simulink model "p4_model"  (R2025b)
settings: Solver=VariableStepAuto  StartTime=0.0  StopTime=10.0  RelTol=1e-3
undefined symbols (not defined in the file or in its folder): carData, datBat, datCar, datMotor
libraries: autolibshared x1, slpidlib x1
(part 3 of 3)

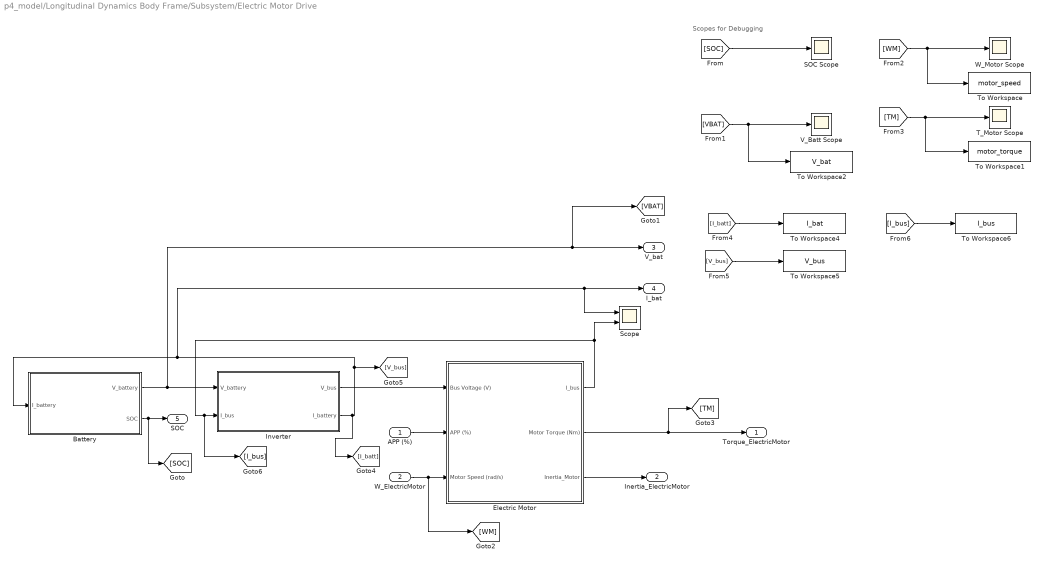
== system p4_model/Longitudinal Dynamics Body Frame/Subsystem/Electric Motor Drive ==
  note: Scopes for Debugging
  APP (%) : Inport
  W_ElectricMotor : Inport  Port=2
  Battery : Subsystem
  Electric Motor : Subsystem
  Inverter : Subsystem
  SOC Scope : Scope
      settings: ActiveDisplayYMinimum=0.79068  ActiveDisplayYMaximum=0.80103  DataLoggingVariableName=ScopeData7
  Scope : Scope  NumInputPorts=2
      settings: ActiveDisplayYMinimum=-92.41521  ActiveDisplayYMaximum=118.26537  DataLoggingVariableName=ScopeData2
  T_Motor Scope : Scope
      settings: ActiveDisplayYMinimum=-92.74121  ActiveDisplayYMaximum=115.47111  DataLoggingVariableName=ScopeData10
  To Workspace : ToWorkspace  VariableName=motor_speed  SaveFormat=Timeseries  SampleTime=-1
  To Workspace1 : ToWorkspace  VariableName=motor_torque  SaveFormat=Timeseries  SampleTime=-1
  To Workspace2 : ToWorkspace  VariableName=V_bat  SaveFormat=Timeseries  SampleTime=-1
  To Workspace4 : ToWorkspace  VariableName=I_bat  SaveFormat=Timeseries  SampleTime=-1
  To Workspace5 : ToWorkspace  VariableName=V_bus  SaveFormat=Timeseries  SampleTime=-1
  To Workspace6 : ToWorkspace  VariableName=I_bus  SaveFormat=Timeseries  SampleTime=-1
  V_Batt Scope : Scope
      settings: ActiveDisplayYMinimum=354.15627  ActiveDisplayYMaximum=391.49042  DataLoggingVariableName=ScopeData8
  W_Motor Scope : Scope
      settings: ActiveDisplayYMinimum=-83.74997  ActiveDisplayYMaximum=695.87961  DataLoggingVariableName=ScopeData9
  Torque_ElectricMotor : Outport
  Inertia_ElectricMotor : Outport  Port=2
  V_bat : Outport  Port=3
  I_bat : Outport  Port=4
  SOC : Outport  Port=5
  wires:
  APP (%)/1 -> Electric Motor/2(APP (%))
  W_ElectricMotor/1 -> [WM], Electric Motor/3(Motor Speed (rad/s))
  Electric Motor/3(Inertia_Motor) -> Inertia_ElectricMotor/1
  Inverter/1(V_bus) -> Electric Motor/1(Bus Voltage (V))
  Inverter/2(I_battery) -> [I_batt], Scope/1, I_bat/1, Battery/1(I_battery), [V_bus]
  Electric Motor/1(I_bus) -> Scope/2, [I_bus], Inverter/2(I_bus)
  [SOC] -> SOC Scope/1
  [VBAT] -> To Workspace2/1, V_Batt Scope/1
  [WM] -> To Workspace/1, W_Motor Scope/1
  [TM] -> To Workspace1/1, T_Motor Scope/1
  Battery/1(V_battery) -> [VBAT], V_bat/1, Inverter/1(V_battery)
  Electric Motor/2(Motor Torque (Nm)) -> [TM], Torque_ElectricMotor/1
  Battery/2(SOC) -> [SOC], SOC/1
  [I_batt] -> To Workspace4/1
  [V_bus] -> To Workspace5/1
  [I_bus] -> To Workspace6/1

== system p4_model/Longitudinal Dynamics Body Frame/Vehicle/vehicleDragForce ==
  vel : Inport
  Drag Force : MATLAB Function  TreatAsAtomicUnit=on
  To Workspace : ToWorkspace  VariableName=Faero  SaveFormat=Timeseries  SampleTime=-1
  drag coeff : Constant  Value=datCar.C2
  rolling friction coeff : Constant  Value=datCar.C1
  static friction : Constant  Value=datCar.C0
  Fdrag : Outport
  wires:
  static friction/1 -> Drag Force/1(C0)
  Drag Force/1(Fdrag) -> Fdrag/1, To Workspace/1
  vel/1 -> Drag Force/4(vel)
  rolling friction coeff/1 -> Drag Force/2(C1)
  drag coeff/1 -> Drag Force/3(C2)

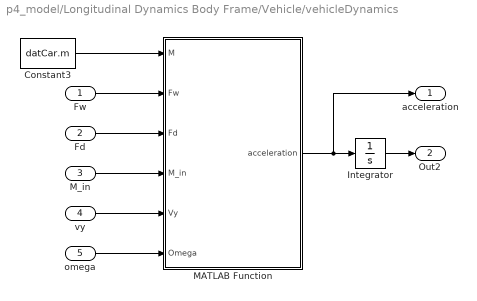
== system p4_model/Longitudinal Dynamics Body Frame/Vehicle/vehicleDynamics ==
  "Fw " : Inport
  Fd : Inport  Port=2
  "M_in " : Inport  Port=3
  vy : Inport  Port=4
  omega : Inport  Port=5
  Constant3 : Constant  Value=datCar.m
  Integrator : Integrator  InitialCondition=datCar.init.vx0  LimitOutput=on  LowerSaturationLimit=0
  MATLAB Function : MATLAB Function  TreatAsAtomicUnit=on
  acceleration : Outport
  Out2 : Outport  Port=2
  wires:
  MATLAB Function/1(acceleration) -> acceleration/1, Integrator/1
  "Fw "/1 -> MATLAB Function/2(Fw)
  vy/1 -> MATLAB Function/5(Vy)
  "M_in "/1 -> MATLAB Function/4(M_in)
  Constant3/1 -> MATLAB Function/1(M)
  omega/1 -> MATLAB Function/6(Omega)
  Fd/1 -> MATLAB Function/3(Fd)
  Integrator/1 -> Out2/1

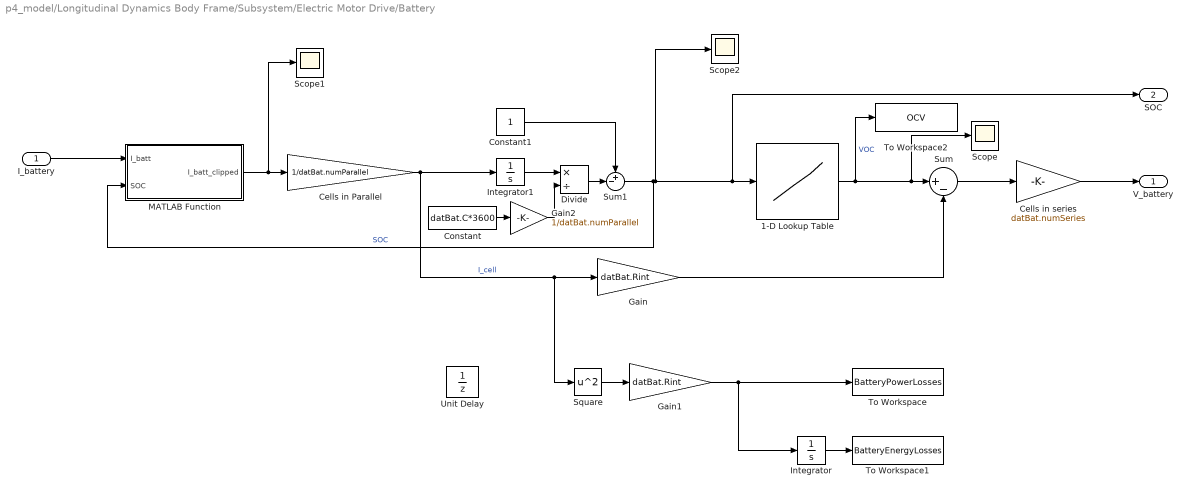
== system p4_model/Longitudinal Dynamics Body Frame/Subsystem/Electric Motor Drive/Battery ==
  I_battery : Inport
  1-D Lookup Table : Lookup_n-D  NumberOfTableDimensions=1  BreakpointsForDimension1=datBat.SOC  Table=datBat.OCV  ExtrapMethod=Clip  UseLastTableValue=on  InternalRulePriority=Speed  RndMeth=Simplest
  Cells in Parallel : Gain  Gain=1/datBat.numParallel
  Cells in series : Gain  Gain=datBat.numSeries
  Constant : Constant  Value=datBat.C*3600
  Constant1 : Constant
  Divide : Product  Inputs=*/
  Gain : Gain  Gain=datBat.Rint
  Gain1 : Gain  Gain=datBat.Rint
  Gain2 : Gain  Gain=1/datBat.numParallel
  Integrator : Integrator
  Integrator1 : Integrator  InitialCondition=1459.5
  MATLAB Function : MATLAB Function  TreatAsAtomicUnit=on
  Scope : Scope
      settings: ActiveDisplayYMinimum=3.9447746248567759  ActiveDisplayYMaximum=3.9505775108183836  DataLoggingVariableName=ScopeData5
  Scope1 : Scope
      settings: ActiveDisplayYMinimum=-38.071970075878966  ActiveDisplayYMaximum=120.71055450400272  DataLoggingVariableName=ScopeData6
  Scope2 : Scope
      settings: ActiveDisplayYMinimum=0.78954924829198925  ActiveDisplayYMaximum=0.80115502179471731
  Square : Math  Operator=square
  Sum : Sum  Inputs=|+-
  Sum1 : Sum  Inputs=+-|
  To Workspace : ToWorkspace  VariableName=BatteryPowerLosses  SaveFormat=Timeseries  SampleTime=-1
  To Workspace1 : ToWorkspace  VariableName=BatteryEnergyLosses  SaveFormat=Timeseries  SampleTime=-1
  To Workspace2 : ToWorkspace  VariableName=OCV  SaveFormat=Timeseries  SampleTime=-1
  Unit Delay : UnitDelay  SampleTime=-1  HasFrameUpgradeWarning=on
  V_battery : Outport
  SOC : Outport  Port=2
  wires:
  Cells in Parallel/1 -> Square/1, Gain/1, Integrator1/1  "I_cell"
  Sum1/1 -> MATLAB Function/2(SOC), Scope2/1, SOC/1, 1-D Lookup Table/1  "SOC"
  1-D Lookup Table/1 -> To Workspace2/1, Scope/1, Sum/1  "VOC"
  Gain/1 -> Sum/2
  Sum/1 -> Cells in series/1
  Cells in series/1 -> V_battery/1
  Integrator1/1 -> Divide/1
  Divide/1 -> Sum1/2
  Constant1/1 -> Sum1/1
  Square/1 -> Gain1/1
  Gain1/1 -> Integrator/1, To Workspace/1
  Integrator/1 -> To Workspace1/1
  Constant/1 -> Gain2/1
  Gain2/1 -> Divide/2
  I_battery/1 -> MATLAB Function/1(I_batt)
  MATLAB Function/1(I_batt_clipped) -> Scope1/1, Cells in Parallel/1

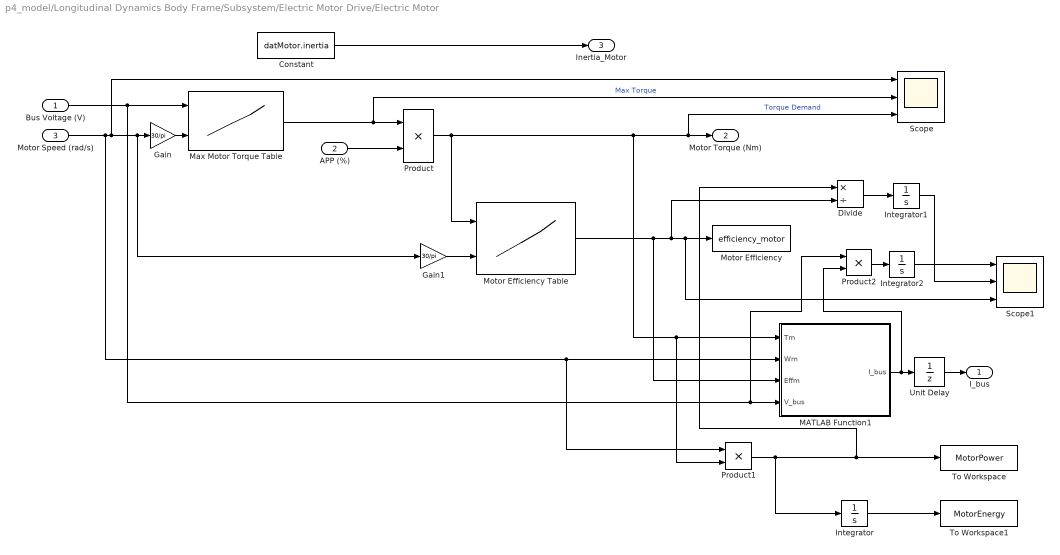
== system p4_model/Longitudinal Dynamics Body Frame/Subsystem/Electric Motor Drive/Electric Motor ==
  Bus Voltage (V) : Inport
  APP (%) : Inport  Port=2
  Motor Speed (rad/s) : Inport  Port=3
  Constant : Constant  Value=datMotor.inertia
  Divide : Product  Inputs=*/
  Gain : Gain  Gain=30/pi
  Gain1 : Gain  Gain=30/pi
  Integrator : Integrator
  Integrator1 : Integrator
  Integrator2 : Integrator
  MATLAB Function1 : MATLAB Function  TreatAsAtomicUnit=on
  Max Motor Torque Table : Lookup_n-D  BreakpointsForDimension1=datMotor.vbus  BreakpointsForDimension2=datMotor.rpm  BreakpointsForDimension3=[5, 7]  Table=datMotor.maxtorque  ExtrapMethod=Clip  UseLastTableValue=on  InternalRulePriority=Speed  RndMeth=Simplest
      settings: InputPortMap=u0,u1
  Motor Efficiency : ToWorkspace  VariableName=efficiency_motor  SaveFormat=Timeseries  SampleTime=-1
  Motor Efficiency Table : Lookup_n-D  BreakpointsForDimension1=datMotor.eta_torque  BreakpointsForDimension2=datMotor.eta_speed  BreakpointsForDimension3=[5, 7]  Table=datMotor.eta_val  ExtrapMethod=Clip  UseLastTableValue=on  InternalRulePriority=Speed  RndMeth=Simplest
      settings: InputPortMap=u0,u1
  Product : Product
  Product1 : Product
  Product2 : Product
  Scope : Scope  NumInputPorts=3
      settings: ActiveDisplayYMinimum=-117.53104  ActiveDisplayYMaximum=699.63306
  Scope1 : Scope  NumInputPorts=3
      settings: ActiveDisplayYMinimum=7.0930778838839177E+6  ActiveDisplayYMaximum=7.1041133971085055E+6  DataLoggingVariableName=ScopeData2
  To Workspace : ToWorkspace  VariableName=MotorPower  SaveFormat=Timeseries  SampleTime=-1
  To Workspace1 : ToWorkspace  VariableName=MotorEnergy  SaveFormat=Timeseries  SampleTime=-1
  Unit Delay : UnitDelay  SampleTime=-1  HasFrameUpgradeWarning=on
  I_bus : Outport
  Motor Torque (Nm) : Outport  Port=2
  Inertia_Motor : Outport  Port=3
  wires:
  Max Motor Torque Table/1 -> Scope/2, Product/1  "Max Torque"
  Constant/1 -> Inertia_Motor/1
  APP (%)/1 -> Product/2
  Product/1 -> Product1/2, MATLAB Function1/1(Tm), Scope/3, Motor Torque (Nm)/1, Motor Efficiency Table/1  "Torque Demand"
  Motor Efficiency Table/1 -> Divide/2, Scope1/3, Motor Efficiency/1, MATLAB Function1/3(Effm)
  MATLAB Function1/1(I_bus) -> Product2/2, Unit Delay/1
  Bus Voltage (V)/1 -> Product2/1, MATLAB Function1/4(V_bus), Max Motor Torque Table/1
  Unit Delay/1 -> I_bus/1
  Product1/1 -> Integrator/1, Divide/1, To Workspace/1
  Integrator/1 -> To Workspace1/1
  Gain/1 -> Max Motor Torque Table/2
  Gain1/1 -> Motor Efficiency Table/2
  Motor Speed (rad/s)/1 -> Product1/1, MATLAB Function1/2(Wm), Scope/1, Gain1/1, Gain/1
  Product2/1 -> Integrator2/1
  Divide/1 -> Integrator1/1
  Integrator1/1 -> Scope1/2
  Integrator2/1 -> Scope1/1

== system p4_model/Longitudinal Dynamics Body Frame/Subsystem/Electric Motor Drive/Inverter ==
  V_battery : Inport
  I_bus : Inport  Port=2
  Efficiency Inverter : Constant  Value=0.95
  Inverter Calculations : MATLAB Function  TreatAsAtomicUnit=on
  V_bus : Outport
  I_battery : Outport  Port=2
  wires:
  V_battery/1 -> Inverter Calculations/1(V_bat)
  Inverter Calculations/1(V_bus) -> V_bus/1
  Efficiency Inverter/1 -> Inverter Calculations/2(Eff_I)
  I_bus/1 -> Inverter Calculations/3(I_bus)
  Inverter Calculations/2(I_bat) -> I_battery/1

== matlab function p4_model/Longitudinal Dynamics Body Frame/Vehicle/vehicleDragForce/Drag Force ==
  data: C0 input; Fdrag output; C1 input; C2 input; vel input
function Fdrag = drag(C0, C1, C2, vel)
    
Fdrag = C0 + C1*vel + C2*(vel)^2;

== matlab function p4_model/Longitudinal Dynamics Body Frame/Vehicle/vehicleDynamics/MATLAB Function ==
  data: M input; Fw input; Fd input; acceleration output; M_in input; Vy input; Omega input
function acceleration = vehicle(M, Fw, Fd, M_in, Vy, Omega)

acceleration = ((Fw - Fd) / (M + M_in)) + Vy*Omega;

== matlab function p4_model/Throttle and Braking Logic /MATLAB Function ==
  data: a input; APP output; b input; v input; BPP output; SOC input; regen output
function [APP, BPP, regen] = fcn(a, b, v, SOC)

    speed1 = 5*1600/3600;
    speed2 = 25*1600/3600;
    dspeed = speed2 - speed1;

    absv = abs(v);
    if absv < speed1
        regen = 0;
    elseif absv <= speed2
        regen = 0.95 * (absv-speed1)/dspeed;
    else
        regen = 0.95;
    end

    if SOC <= 0.8
        SOCfactor = 1;
    elseif SOC < 1
        SOCfactor = 1 - (SOC-0.8)/(1-0.8);
    else
        SOCfactor = 0;
    end

    regen = regen * SOCfactor;

    APP = a + b*regen;
    BPP = b * (1-regen);
    %APP=a;
    %BPP=b;

== matlab function p4_model/Longitudinal Dynamics Body Frame/Subsystem/Electric Motor Drive/Battery/MATLAB Function ==
  data: I_batt input; SOC input; I_batt_clipped output
function I_batt_clipped = fcn(I_batt, SOC)
    if SOC <= 0.1
        I_batt_clipped = 0;
    else
        I_batt_clipped = I_batt;
    end

== matlab function p4_model/Throttle and Braking Logic /MATLAB Function1 ==
  data: regen input; viol output; v input
function viol = fcn(regen, v)
    if v < (5*(1600/3600))
        regen_vio = 0;
        if regen == regen_vio
            viol = 0;
        else
            viol = 1;
        end

    elseif v == (25*(1600/3600))
        regen_vio = 0.95;
        if regen == regen_vio
            viol = 0;
        else
            viol = 1;
        end

    elseif v > (25*(1600/3600))
        regen_vio = 0.95;
        if regen == regen_vio
            viol = 0;
        else
            viol = 1;
        end
    else
        regen_vio = (0.95/20)*v;
        if regen == regen_vio
            viol = 0;
        else
            viol = 1;
        end
    end

%     BRK = BPP * -1;
%     if(BRK >= 0) && (1 >= BRK)
%         viol = 0;
%     else
%         viol = 1;
%     end

== matlab function p4_model/CarLateralKinematicsModelBodyFrame/Tire Slip ==
  data: alpha_r output; vy input; alpha_f output; vx input; delta_f input; omega input; obj input
function [alpha_r, alpha_f] = fcn(vy, vx, delta_f, omega, obj)
    % obj must provide: vx_threshold1, lf, lr

    if abs(vx) > obj.vx_threshold1
        alpha_f = delta_f - (vy + omega .* obj.lf) ./ vx;
        alpha_r = - (vy - omega .* obj.lr) ./ vx;
    else
        alpha_f = 0;
        alpha_r = 0;
    end
end

== matlab function p4_model/CarLateralKinematicsModelBodyFrame/Tire Forces ==
  data: Fyr output; Fyf output; alpha_r input; alpha_f input; obj input
function [Fyr, Fyf] = fcn(alpha_r, alpha_f, obj)
    % obj must have fields/properties: Calpha_r, Calpha_f, Fyrmax, Fyfmax

    Fyr = obj.Calpha_r .* alpha_r;
    Fyf = obj.Calpha_f .* alpha_f;

    % clamp to ±Fyrmax and ±Fyfmax
    Fyr = max(-obj.Fyrmax, min(obj.Fyrmax, Fyr));
    Fyf = max(-obj.Fyfmax, min(obj.Fyfmax, Fyf));
end

== matlab function p4_model/CarBodyFrame2InertialFrame/KinematicVehicleModel_derivatives ==
  data: vx input; vy input; psi input size=1; Xdot output; Ydot output
function [Xdot, Ydot] = fcn(vx, vy, psi)
    temp = TF(psi) * [vx; vy];
    Xdot = temp(1);
    Ydot = temp(2);
end

function R = TF(psi)
    R = [cos(psi), -sin(psi); sin(psi), cos(psi)];
end

== matlab function p4_model/CarLateralKinematicsModelBodyFrame/Lateral Dynamics ==
  data: Fyr input; ay output; Fyf input; vx input; omega input; omega_dot output; obj input
function [ay, omega_dot] = fcn(Fyr, Fyf, vx, omega, obj)
    % obj must have fields/properties: Mass, Inertia, lf, lr
    ay = -vx.*omega + (Fyf + Fyr)./obj.Mass;
    omega_dot = (Fyf.*obj.lf - Fyr.*obj.lr)./obj.Inertia;
end

== matlab function p4_model/Longitudinal Dynamics Body Frame/Subsystem/Electric Motor Drive/Electric Motor/MATLAB Function1 ==
  data: Tm input; I_bus output; Wm input; Effm input; V_bus input
function I_bus = fcn(Tm, Wm, Effm, V_bus)
    Pm = Tm*Wm;
    sgn_m = Pm / (abs(Pm) + 0.001);
    Pe = Pm / (Effm^sgn_m);
    if V_bus > 1
        I_bus = Pe/V_bus;
    else
        I_bus = 0;
    end

== matlab function p4_model/Longitudinal Dynamics Body Frame/Subsystem/Electric Motor Drive/Inverter/Inverter Calculations ==
  data: V_bat input; Eff_I input; V_bus output; I_bus input; I_bat output
function [V_bus, I_bat] = fcn(V_bat, Eff_I, I_bus)
    V_bus = V_bat; % Vbus = Vbat * r, where r is the inverter conversion ratio % * I_bat * Eff_I^(sgn_Pbat))/ I_bus;
    P_bus = V_bus *I_bus;
    sgn_Pbus = P_bus / (abs(P_bus) + 0.001);
    
    if V_bat > 1
        I_bat = (P_bus / Eff_I^sgn_Pbus) / V_bat ;
    else
        I_bat = 0;
    end

end

% double check

== matlab function p4_model/Friction ==
  data: BPP_total input; BPP_friction output; v_mps input; BPP_regen output
function [BPP_friction, BPP_regen] = fcn(BPP_total, v_mps)
    mph2mps = 0.44704;
    v_mph   = v_mps / mph2mps;

    if v_mph < 5
        min_fric_frac = 1.0;
    elseif v_mph <= 25
        min_fric_frac = 1.0 - 0.95 * (v_mph - 5) / 20;
    else
        min_fric_frac = 0.05;
    end

    BPP_friction = BPP_total * min_fric_frac;
    BPP_regen    = BPP_total * (1 - min_fric_frac);
end

== matlab function p4_model/Driver/MATLAB Function ==
  data: X input; Y input; psi_int input; psi input; omega input; delta_f output; vx output; obj input
function [delta_f, vx] = SimplestDriver(X, Y, psi_int, psi, omega, obj)
% PD + feedforward steering controller for oval track

% --- track geometry ---
R   = 200;      % radius of curves (m)
Lst = 900;      % length of straights (m)
cy  = R;        % y-coordinate of both curve centers

% --- controller gains ---
Kp = 0.5;     % proportional gain on heading error (rad/rad)
Ki = 0;       % integral gain (psi_int input is not wired; disabled)
Kd = 2.0;     % derivative gain on yaw-rate error (rad/(rad/s))
maxSteer = 0.5;    % max steering angle (rad)

vx = obj.vxd;      % target longitudinal speed (constant)

% --- reference heading and curvature from vehicle position ---
% Both curves are counterclockwise (center is always to the left of travel),
% so kappa_ref = +1/R for both.
if X > Lst
    % Right semicircle: center at (Lst, cy)
    phi       = atan2(Y - cy, X - Lst);
    psi_ref   = phi + pi/2;
    kappa_ref = 1/R;
elseif X < 0
    % Left semicircle: center at (0, cy)
    phi       = atan2(Y - cy, X);
    psi_ref   = phi + pi/2;
    kappa_ref = 1/R;    % also counterclockwise: west->south->east
else
    % Straight sections: use Y position to pick which straight
    kappa_ref = 0;
    if Y < cy
        psi_ref = 0;     % bottom straight: heading east  (+x)
    else
        psi_ref = pi;    % top straight:    heading west  (-x)
    end
end

% --- feedforward: Ackermann geometry ---
delta_ff = (obj.lf + obj.lr) * kappa_ref;

% --- heading error wrapped to [-pi, pi] ---
e_psi = wrapToPi(psi_ref - psi);

% --- yaw-rate reference from curvature ---
omega_ref = kappa_ref * vx;

% --- PD control law ---
delta = delta_ff + Kp*e_psi + Ki*psi_int - Kd*(omega - omega_ref);

% --- saturate steering ---
delta_f = min(max(delta, -maxSteer), maxSteer);
end
